simulink model "inverter"  (R2024b)
settings: Solver=VariableStepAuto  StartTime=0.0  StopTime=0.5  RelTol=1e-3
libraries: spsIGBTDiodeLib x6, spsDCVoltageSourceLib x1, spsGroundLib x1, spsThreePhaseParallelRLCBranchLib x1, spsThreePhaseVIMeasurementLib x1, sps_lib x1
settings Model: Creator=ETC  LastModifiedBy=ETC

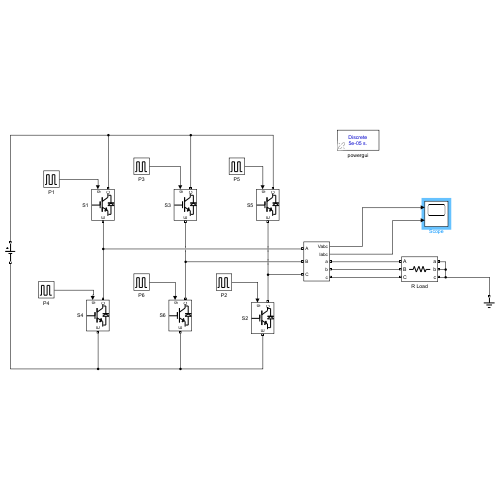
[thumbnail: Simulink's stored preview of the top-level diagram]
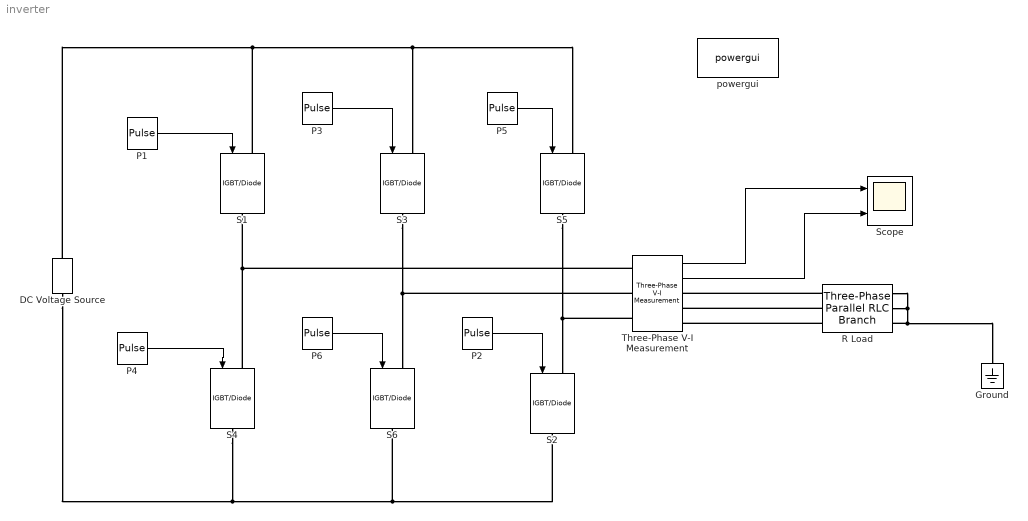
== system inverter ==
  DC Voltage Source : spsDCVoltageSourceLib/DC Voltage Source  Amplitude=400  Measurements=None
  Ground : spsGroundLib/Ground  LConnTagsString=a
  P1 : DiscretePulseGenerator  PulseType=Time based  Period=0.02  PulseWidth=50  PhaseDelay=0*0.02/360
  P2 : DiscretePulseGenerator  PulseType=Time based  Period=0.02  PulseWidth=50  PhaseDelay=60*0.02/360
  P3 : DiscretePulseGenerator  PulseType=Time based  Period=0.02  PulseWidth=50  PhaseDelay=120*0.02/360
  P4 : DiscretePulseGenerator  PulseType=Time based  Period=0.02  PulseWidth=50  PhaseDelay=180*0.02/360
  P5 : DiscretePulseGenerator  PulseType=Time based  Period=0.02  PulseWidth=50  PhaseDelay=240*0.02/360
  P6 : DiscretePulseGenerator  PulseType=Time based  Period=0.02  PulseWidth=50  PhaseDelay=300*0.02/360
  R Load : spsThreePhaseParallelRLCBranchLib/Three-Phase Parallel RLC Branch  LConnTagsString=A|B|C  RConnTagsString=A|B|C  BranchType=R  Resistance=1  Inductance=1e-3  Capacitance=1e-6  Measurements=None
  S{1..6} (6 alike) : spsIGBTDiodeLib/IGBT//Diode  Ron=1e-3  Rs=1e5  Cs=inf  Measurements=off
  Scope : Scope  NumInputPorts=2
  Three-Phase V-I Measurement : spsThreePhaseVIMeasurementLib/Three-Phase V-I Measurement  VoltageMeasurement=phase-to-ground  SetLabelV=off  LabelV=Vabc  Vpu=off  VpuLL=off  CurrentMeasurement=yes  SetLabelI=off  LabelI=Iabc  Ipu=off  Pbase=100e6  Vbase=500e3  OutputType=Complex  PhasorSimulation=off  PSBequivalent=0
  powergui : sps_lib/powergui  Priority=1  SimulationMode=Discrete  SampleTime=50e-6  frequency=60  Iterations=50  frequencyindice=0  Pbase=100e6  ErrMax=1e-4  UnitsV=kV  UnitsW=MW  buscounter=0  FunctionMessages=off  echomessages=off  EnableUseOfTLC=off  CurrentSourceSwitches=off  DisableSnubberDevices=off  DisableRonSwitches=off  DisableVfSwitches=off  DisplayEquations=off  AutomaticDiscreteSolvers=off  SolverType=Tustin/Backward Euler (TBE)  Interpol=off  ExternalGateDelay=off  methode=off  Ts=100  x0status=blocks  SPID=on  SwTol=0  HookPort=off  NonlinearTolerance=1e-4  nMaxIteration=100  ContinueOnMaxIteration=off  RestoreLinks=warning  ResistiveCurrentMeasurement=off  Frange=[0:2:500]  Ylog=off  Xlog=on  ShowGrid=off  save=off  variable=ZData  structure=0  ZoomFFT=off  StartTime=0.0  cycles=1  DisplayStyle=1  fundamental=60  FreqAxis=off  MaxFrequency=1000  frequencyindicesteady=1  RmsSteady=1  display=off
  wires:
  P1/1 -> S1/1
  P2/1 -> S2/1
  P3/1 -> S3/1
  P4/1 -> S4/1
  P5/1 -> S5/1
  P6/1 -> S6/1
  Three-Phase V-I Measurement/1 -> Scope/1
  Three-Phase V-I Measurement/2 -> Scope/2
  connections:
  S4/LConn1 -- S1/RConn1 -- Three-Phase V-I Measurement/LConn1
  S3/RConn1 -- Three-Phase V-I Measurement/LConn2 -- S6/LConn1
  S5/RConn1 -- Three-Phase V-I Measurement/LConn3 -- S2/LConn1
  S1/LConn1 -- DC Voltage Source/RConn1 -- S3/LConn1 -- S5/LConn1
  S4/RConn1 -- DC Voltage Source/LConn1 -- S6/RConn1 -- S2/RConn1
  R Load/LConn1 -- Three-Phase V-I Measurement/RConn1
  R Load/LConn2 -- Three-Phase V-I Measurement/RConn2
  R Load/LConn3 -- Three-Phase V-I Measurement/RConn3
  R Load/RConn1 -- R Load/RConn2 -- Ground/LConn1 -- R Load/RConn3
